simulink model "rahcel_pump_vs_pd_pump"  (R2025b)
settings: Solver=VariableStepAuto  StartTime=0.0  StopTime=0.1  RelTol=1e-3
values from neighbouring files (symbols this model uses):
  param = struct()    [Copy_of_param_file.m]    (also in param_file.m; param_file_loss_vs_freq.m; param_file_original.m; param_file_turbine.m)
settings Model: Creator=user  LastModifiedBy=mahmu

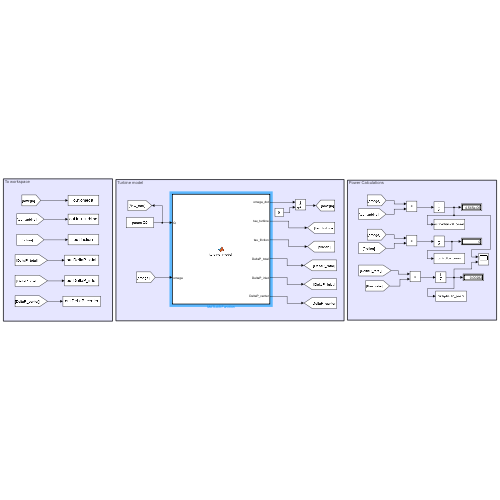
[thumbnail: Simulink's stored preview of the top-level diagram]
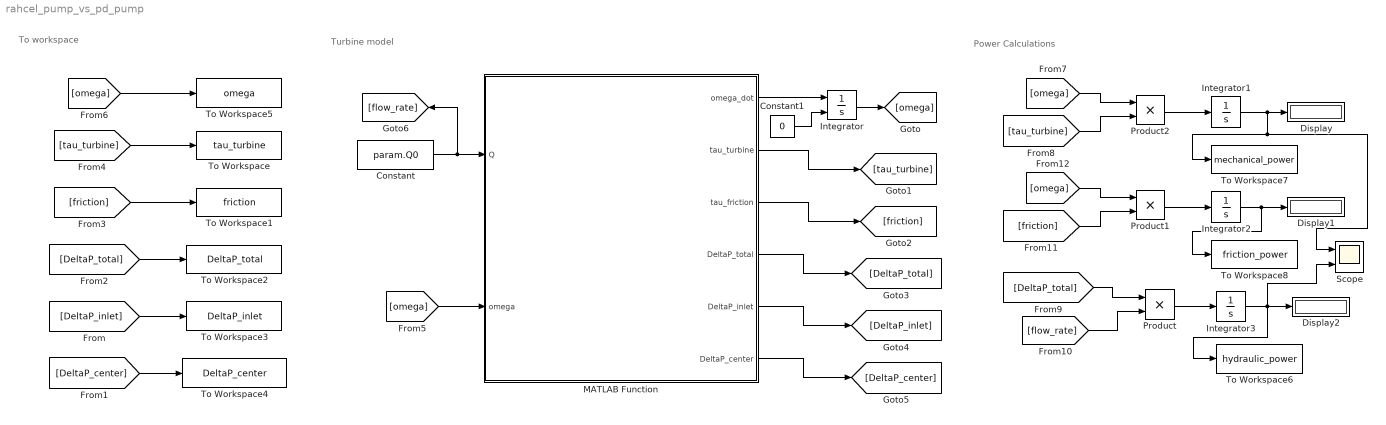
== system rahcel_pump_vs_pd_pump ==
  note: Power Calculations
  note: Turbine model
  note: To workspace
  Constant : Constant  Value=param.Q0
  Constant1 : Constant  Value=0
  Display : Display
  Display1 : Display
  Display2 : Display
  Integrator : Integrator  InitialConditionSource=external
  Integrator1 : Integrator
  Integrator2 : Integrator
  Integrator3 : Integrator
  MATLAB Function : MATLAB Function  TreatAsAtomicUnit=on
  Product : Product
  Product1 : Product
  Product2 : Product
  Scope : Scope  NumInputPorts=2
      settings: ActiveDisplayYMinimum=-1.0287117188973947E-5  ActiveDisplayYMaximum=3.4847493314143685E-5
  To Workspace : ToWorkspace  VariableName=tau_turbine  SaveFormat=Timeseries  SampleTime=-1
  To Workspace1 : ToWorkspace  VariableName=friction  SaveFormat=Timeseries  SampleTime=-1
  To Workspace2 : ToWorkspace  VariableName=DeltaP_total  SaveFormat=Timeseries  SampleTime=-1
  To Workspace3 : ToWorkspace  VariableName=DeltaP_inlet  SaveFormat=Timeseries  SampleTime=-1
  To Workspace4 : ToWorkspace  VariableName=DeltaP_center  SaveFormat=Timeseries  SampleTime=-1
  To Workspace5 : ToWorkspace  VariableName=omega  SaveFormat=Timeseries  SampleTime=-1
  To Workspace6 : ToWorkspace  VariableName=hydraulic_power  SaveFormat=Timeseries  SampleTime=-1
  To Workspace7 : ToWorkspace  VariableName=mechanical_power  SaveFormat=Timeseries  SampleTime=-1
  To Workspace8 : ToWorkspace  VariableName=friction_power  SaveFormat=Timeseries  SampleTime=-1
  wires:
  MATLAB Function/1(omega_dot) -> Integrator/1
  Integrator/1 -> [omega]
  Constant/1 -> MATLAB Function/1(Q), [flow_rate]
  MATLAB Function/2(tau_turbine) -> [tau_turbine]
  MATLAB Function/3(tau_friction) -> [friction]
  MATLAB Function/4(DeltaP_total) -> [DeltaP_total]
  MATLAB Function/5(DeltaP_inlet) -> [DeltaP_inlet]
  MATLAB Function/6(DeltaP_center) -> [DeltaP_center]
  [DeltaP_center] -> To Workspace4/1
  [DeltaP_inlet] -> To Workspace3/1
  [DeltaP_total] -> To Workspace2/1
  [friction] -> To Workspace1/1
  [tau_turbine] -> To Workspace/1
  [omega] -> MATLAB Function/2(omega)
  [omega] -> To Workspace5/1
  [DeltaP_total] -> Product/1
  [flow_rate] -> Product/2
  [omega] -> Product1/1
  [friction] -> Product1/2
  [omega] -> Product2/1
  [tau_turbine] -> Product2/2
  Constant1/1 -> Integrator/2
  Product2/1 -> Integrator1/1
  Product1/1 -> Integrator2/1
  Integrator1/1 -> Scope/1, To Workspace7/1, Display/1
  Integrator2/1 -> To Workspace8/1, Display1/1
  Integrator3/1 -> Scope/2, To Workspace6/1, Display2/1
  Product/1 -> Integrator3/1

== matlab function rahcel_pump_vs_pd_pump/MATLAB Function ==
  data: Q input; omega_dot output; omega input; tau_turbine output; tau_friction output; DeltaP_total output; DeltaP_inlet output; DeltaP_center output; param parameter
function [omega_dot, tau_turbine, tau_friction, DeltaP_total, DeltaP_inlet, DeltaP_center] = turbine_model(Q, omega, param)

% Make sure flow is positive
Q_eff = max(Q, 0);

% Turbine torque
tau_turbine = (param.rho*param.R_in/(param.A_in*param.N))*Q_eff^2;

% Friction torque
% tau_friction = param.A_surf*(param.mu*param.R^2/(param.c + param.eps_val))*omega;
tau_friction = 0;

% Rotor dynamics
omega_dot = (tau_turbine - tau_friction)/(param.J + param.eps_val);

% Pressure drop
DeltaP_inlet = (param.rho/2)*(Q_eff/(param.Cd_in*param.A_rhombus + param.eps_val))^2;

% DeltaP_center = Q_eff^param.m/(param.k_center*param.D^param.n + param.eps_val);
DeltaP_center = 0;

DeltaP_total = DeltaP_inlet + DeltaP_center;

end
